simulink library "INT_FlSys_CalcCnvFac"  (R2016b)
settings: Solver=VariableStepAuto  StartTime=0.0  StopTime=10.0  RelTol=1e-3
settings Model: Creator=Administrator  LastModifiedBy=Administrator

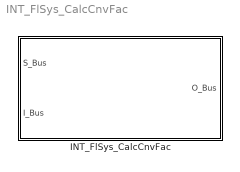
== system INT_FlSys_CalcCnvFac ==
  INT_FlSys_CalcCnvFac : Subsystem

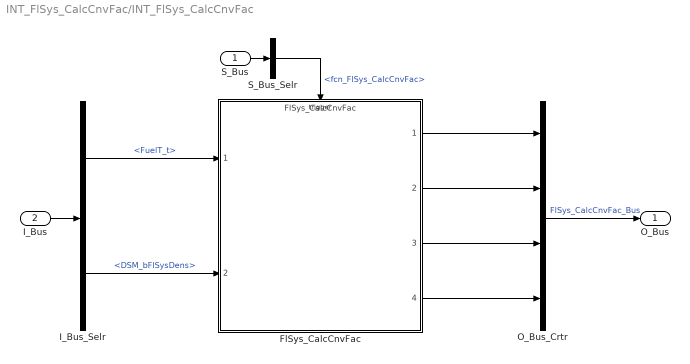
== system INT_FlSys_CalcCnvFac/INT_FlSys_CalcCnvFac ==
  S_Bus : Inport
  I_Bus : Inport  Port=2
  FlSys_CalcCnvFac : ModelReference  ModelNameDialog=FlSys_CalcCnvFac  SimulationMode=Normal  ModelReferenceVersion=1.9  TriggerPortName=function  TriggerPortTriggerType=function-call  TriggerPortStatesWhenEnabling=held
  I_Bus_Selr : BusSelector  OutputSignals=FuelT_t,DSM_bFlSysDens
  O_Bus_Crtr : BusCreator  Inputs=4
  S_Bus_Selr : BusSelector  OutputSignals=fcn_FlSys_CalcCnvFac
  O_Bus : Outport
  wires:
  S_Bus_Selr/1 -> FlSys_CalcCnvFac/Trigger  "<fcn_FlSys_CalcCnvFac>"
  S_Bus/1 -> S_Bus_Selr/1
  I_Bus/1 -> I_Bus_Selr/1
  I_Bus_Selr/1 -> FlSys_CalcCnvFac/1  "<FuelT_t>"
  I_Bus_Selr/2 -> FlSys_CalcCnvFac/2  "<DSM_bFlSysDens>"
  O_Bus_Crtr/1 -> O_Bus/1  "FlSys_CalcCnvFac_Bus"
  FlSys_CalcCnvFac/1 -> O_Bus_Crtr/1
  FlSys_CalcCnvFac/2 -> O_Bus_Crtr/2
  FlSys_CalcCnvFac/3 -> O_Bus_Crtr/3
  FlSys_CalcCnvFac/4 -> O_Bus_Crtr/4
